simulink model "conv_3_2_2"  (R2013a)
settings: Solver=VariableStepDiscrete  StartTime=0.0  StopTime=10.0  RelTol=1e-3
settings Model: Creator=remiburtin  LastModifiedBy=remiburtin

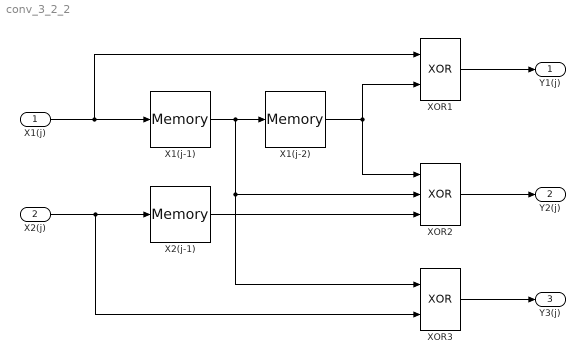
== system conv_3_2_2 ==
  X1(j) : Inport
  X2(j) : Inport  Port=2
  X1(j-1) : Memory
  X1(j-2) : Memory
  X2(j-1) : Memory
  "XOR1 " : Logic  Operator=XOR  AllPortsSameDT=off  OutDataTypeStr=boolean
  XOR2 : Logic  Operator=XOR  Inputs=3  AllPortsSameDT=off  OutDataTypeStr=boolean
  XOR3 : Logic  Operator=XOR  AllPortsSameDT=off  OutDataTypeStr=boolean
  Y1(j) : Outport
  Y2(j) : Outport  Port=2
  Y3(j) : Outport  Port=3
  wires:
  X1(j-1)/1 -> XOR2/2, XOR3/1, X1(j-2)/1
  X1(j-2)/1 -> XOR2/1, "XOR1 "/2
  X2(j-1)/1 -> XOR2/3
  X1(j)/1 -> "XOR1 "/1, X1(j-1)/1
  X2(j)/1 -> XOR3/2, X2(j-1)/1
  "XOR1 "/1 -> Y1(j)/1
  XOR2/1 -> Y2(j)/1
  XOR3/1 -> Y3(j)/1
